simulink model "direction_id"  (R2023a)
settings: configuration reference "config" (kept outside this file)
libraries: simulink x2
settings Model: DataDictionary=model_config.sldd  Creator=huangcheng  LastModifiedBy=Administrator
settings ConfigSetRef: SourceName=config

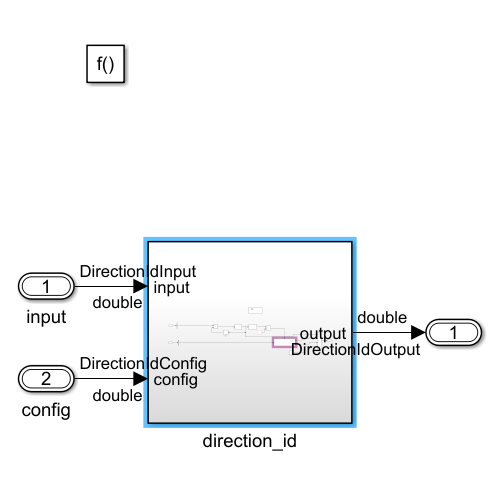
[thumbnail: Simulink's stored preview of the top-level diagram]
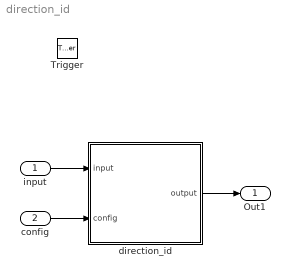
== system direction_id ==
  input : Inport  OutDataTypeStr=Bus: DirectionIdInput  BusOutputAsStruct=on
  config : Inport  Port=2  OutDataTypeStr=Bus: DirectionIdConfig  BusOutputAsStruct=on
  Trigger : TriggerPort  TriggerType=function-call  VariantControl=(inherit)  PortDimensions=1
  direction_id : Subsystem  SystemSampleTime=10e-5
  Out1 : Outport  OutDataTypeStr=Bus: DirectionIdOutput  BusOutputAsStruct=on
  wires:
  direction_id/1(output) -> Out1/1
  input/1 -> direction_id/1(input)
  config/1 -> direction_id/2(config)

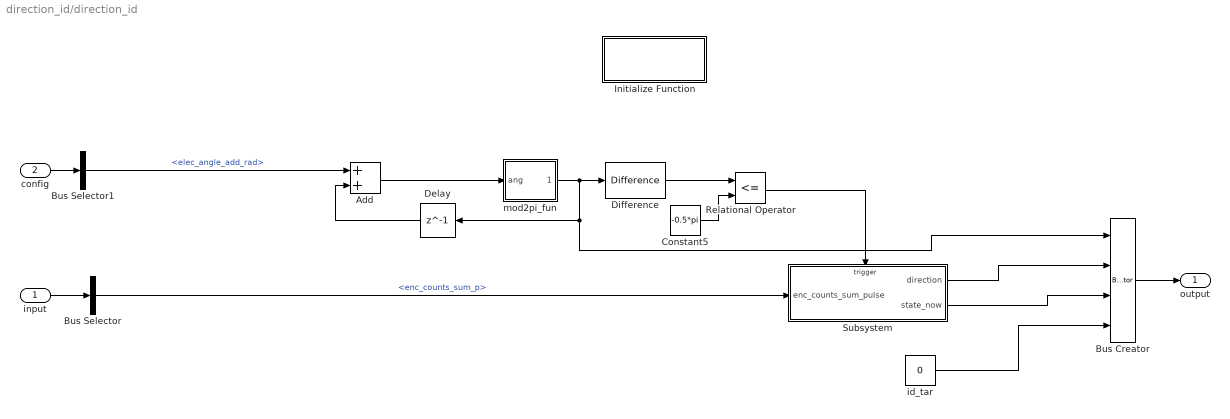
== system direction_id/direction_id ==
  input : Inport
  config : Inport  Port=2
  Add : Sum
  Bus Creator : BusCreator  Inputs=4  OutDataTypeStr=Bus: DirectionIdOutput  NonVirtualBus=on
      settings: InheritFromInputs=off
  Bus Selector : BusSelector  OutputSignals=enc_counts_sum_p
  Bus Selector1 : BusSelector  OutputSignals=elec_angle_add_rad
  Constant5 : Constant  Value=-0.5*pi
  Delay : Delay  DelayLength=1  StateName=elec_angle_tar_last
  Difference : simulink/Discrete/Difference  ICPrevInput=0.0  OutMin=[]  OutMax=[]  OutDataType=fixdt(1, 16)  OutScaling=2^-10  DoSatur=off
  Initialize Function : Subsystem  TreatAsAtomicUnit=on
  Relational Operator : RelationalOperator  Operator=<=  OutDataTypeStr=boolean  RndMeth=Simplest  InputSameDT=off
  Subsystem : Subsystem
  id_tar : Constant  Value=0  OutDataTypeStr=single
  mod2pi_fun : MATLAB Function  TreatAsAtomicUnit=on
  output : Outport
  wires:
  Bus Selector1/1 -> Add/1  "<elec_angle_add_rad>"
  Add/1 -> mod2pi_fun/1(ang)
  Difference/1 -> Relational Operator/1
  Delay/1 -> Add/2
  mod2pi_fun/1(n_ang) -> Bus Creator/1, Delay/1, Difference/1
  Relational Operator/1 -> Subsystem/Trigger
  Constant5/1 -> Relational Operator/2
  Subsystem/1(direction) -> Bus Creator/2
  Subsystem/2(state_now) -> Bus Creator/3
  input/1 -> Bus Selector/1
  config/1 -> Bus Selector1/1
  Bus Selector/1 -> Subsystem/1(enc_counts_sum_pulse)  "<enc_counts_sum_p>"
  Bus Creator/1 -> output/1
  id_tar/1 -> Bus Creator/4

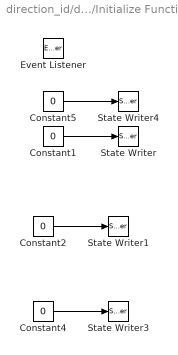
== system direction_id/direction_id/Initialize Function ==
  Constant1 : Constant  Value=0  OutDataTypeStr=single
  Constant2 : Constant  Value=0  OutDataTypeStr=uint8
  Constant4 : Constant  Value=0  OutDataTypeStr=int8
  Constant5 : Constant  Value=0  OutDataTypeStr=boolean
  Event Listener : EventListener  DisableCoverage=on  EventName=reset
  State Writer : StateWriter  StateOwnerBlock=../../Delay  StateName=elec_angle_tar_last
  State Writer1 : StateWriter  StateOwnerBlock=../../Subsystem/Delay2  StateName=step_num
  State Writer3 : StateWriter  StateOwnerBlock=../../Subsystem/state_now
  State Writer4 : StateWriter  StateOwnerBlock=../../Subsystem/Trigger
  wires:
  Constant5/1 -> State Writer4/1
  Constant1/1 -> State Writer/1
  Constant4/1 -> State Writer3/1
  Constant2/1 -> State Writer1/1

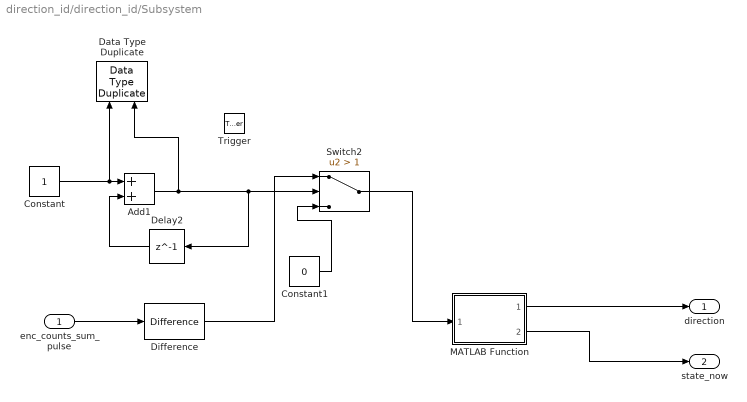
== system direction_id/direction_id/Subsystem ==
  enc_counts_sum_pulse : Inport
  Trigger : TriggerPort  VariantControl=(inherit)  PortDimensions=1
  Add1 : Sum
  Constant : Constant  OutDataTypeStr=uint8
  Constant1 : Constant  Value=0  OutDataTypeStr=int64
  Data Type Duplicate : DataTypeDuplicate
  Delay2 : Delay  DelayLength=1  InitialCondition=0  StateName=step_num
  Difference : simulink/Discrete/Difference  ICPrevInput=0.0  OutMin=[]  OutMax=[]  OutDataType=fixdt(1, 16)  OutScaling=2^-10  DoSatur=off
  MATLAB Function : MATLAB Function  TreatAsAtomicUnit=on
  Switch2 : Switch  Criteria=u2 > Threshold  Threshold=1  SaturateOnIntegerOverflow=off  InputSameDT=off
  direction : Outport
  state_now : Outport  Port=2
  wires:
  enc_counts_sum_pulse/1 -> Difference/1
  MATLAB Function/1(direction) -> direction/1
  MATLAB Function/2(state_now) -> state_now/1
  Constant/1 -> Data Type Duplicate/1, Add1/1
  Delay2/1 -> Add1/2
  Add1/1 -> Switch2/2, Delay2/1, Data Type Duplicate/2
  Difference/1 -> Switch2/1
  Switch2/1 -> MATLAB Function/1(diff_pos)
  Constant1/1 -> Switch2/3

== matlab function direction_id/mod2pi_fun ==
  data: ang input; n_ang output
function n_ang = mod2pi(ang)
    % 将角度限制在0到2π范围内
    TWO_PI = single(2*pi);
    n_ang = single(ang);
    while n_ang < 0
        n_ang = n_ang + TWO_PI;
    end
    while n_ang >= TWO_PI
        n_ang = n_ang - TWO_PI;
    end
end

== matlab function direction_id/Subsystem/MATLAB Function ==
  data: diff_pos input; direction output; state_now output
function [direction, state_now] = direction_id(diff_pos)

if diff_pos > int64(0)
    direction = int8(1);
    state_now = int8(3);
elseif diff_pos < int64(0)
    direction = int8(-1);
    state_now = int8(3);
else
    direction = int8(0);
    state_now = int8(2);
end
